simulink model "QueuingSys"  (R2019a)
settings: Solver=VariableStepAuto  StartTime=0.0  StopTime=100  RelTol=1e-3  EnableMultiTasking=on
undefined symbols (not defined in the file or in its folder): m, n
(part 2 of 5)

== system QueuingSys/Server18 ==
  Entity Generator1 : EntityGenerator  OutputPortMessageModes=m  TimeSource=MATLAB action  IntergenerationTimeAction=dt =MMPPArrivalTime35();  EntityType=Structured  EntityTypeName=Entity
  Entity Queue1 : EntityQueue  InputPortMessageModes=m  OutputPortMessageModes=m  Capacity=Inf  MulticastTag=B
      settings: OutputPortMap=o5
  Entity Server : EntityServer  InputPortMessageModes=m  OutputPortMessageModes=m  Capacity=2  ServiceTimeSource=MATLAB action  ServiceTimeAction=dt =MMPPArrivalTime36();
  OS : EntityOutputSwitch  InputPortMessageModes=m  OutputPortMessageModes=m,m,m,m,m,m,m,m,m,m,m,m,m,m,m,m,m,m,m,m  NumberOutputPorts=20  SwitchingCriterion=Round robin  SwitchAttributeName=Attribute1
      settings: OutputPortMap=o0,o1,o2,o3,o4,o5,o6,o7,o8,o9,o10,o11,o12,o13,o14,o15,o16,o17,o18,o19
  tag scope: Goto18_10=global, Goto18_11=global, Goto18_12=global, Goto18_13=global, Goto18_14=global, Goto18_15=global, Goto18_16=global, Goto18_17=global, Goto18_18=global, Goto18_19=global, Goto18_1=global, Goto18_20=global, Goto18_2=global, Goto18_3=global, Goto18_4=global, Goto18_5=global, Goto18_6=global, Goto18_7=global, Goto18_8=global, Goto18_9=global
  wires:
  Entity Queue1/1 -> Entity Server/1
  Entity Generator1/1 -> Entity Queue1/1
  Entity Server/1 -> OS/1
  OS/1 -> [Goto18_1]
  OS/2 -> [Goto18_2]
  OS/3 -> [Goto18_3]
  OS/4 -> [Goto18_4]
  OS/5 -> [Goto18_5]
  OS/6 -> [Goto18_6]
  OS/7 -> [Goto18_7]
  OS/8 -> [Goto18_8]
  OS/9 -> [Goto18_9]
  OS/10 -> [Goto18_10]
  OS/11 -> [Goto18_11]
  OS/12 -> [Goto18_12]
  OS/13 -> [Goto18_13]
  OS/14 -> [Goto18_14]
  OS/15 -> [Goto18_15]
  OS/16 -> [Goto18_16]
  OS/17 -> [Goto18_17]
  OS/18 -> [Goto18_18]
  OS/19 -> [Goto18_19]
  OS/20 -> [Goto18_20]

== system QueuingSys/Server19 ==
  Entity Generator1 : EntityGenerator  OutputPortMessageModes=m  TimeSource=MATLAB action  IntergenerationTimeAction=dt =MMPPArrivalTime37();  EntityType=Structured  EntityTypeName=Entity
  Entity Queue1 : EntityQueue  InputPortMessageModes=m  OutputPortMessageModes=m  Capacity=Inf  MulticastTag=B
      settings: OutputPortMap=o5
  Entity Server : EntityServer  InputPortMessageModes=m  OutputPortMessageModes=m  Capacity=3  ServiceTimeSource=MATLAB action  ServiceTimeAction=dt =MMPPArrivalTime38();
  OS : EntityOutputSwitch  InputPortMessageModes=m  OutputPortMessageModes=m,m,m,m,m,m,m,m,m,m,m,m,m,m,m,m,m,m,m,m  NumberOutputPorts=20  SwitchingCriterion=Round robin  SwitchAttributeName=Attribute1
      settings: OutputPortMap=o0,o1,o2,o3,o4,o5,o6,o7,o8,o9,o10,o11,o12,o13,o14,o15,o16,o17,o18,o19
  tag scope: Goto19_10=global, Goto19_11=global, Goto19_12=global, Goto19_13=global, Goto19_14=global, Goto19_15=global, Goto19_16=global, Goto19_17=global, Goto19_18=global, Goto19_19=global, Goto19_1=global, Goto19_20=global, Goto19_2=global, Goto19_3=global, Goto19_4=global, Goto19_5=global, Goto19_6=global, Goto19_7=global, Goto19_8=global, Goto19_9=global
  wires:
  Entity Server/1 -> OS/1
  Entity Generator1/1 -> Entity Queue1/1
  Entity Queue1/1 -> Entity Server/1
  OS/1 -> [Goto19_1]
  OS/2 -> [Goto19_2]
  OS/3 -> [Goto19_3]
  OS/4 -> [Goto19_4]
  OS/5 -> [Goto19_5]
  OS/6 -> [Goto19_6]
  OS/7 -> [Goto19_7]
  OS/8 -> [Goto19_8]
  OS/9 -> [Goto19_9]
  OS/10 -> [Goto19_10]
  OS/11 -> [Goto19_11]
  OS/12 -> [Goto19_12]
  OS/13 -> [Goto19_13]
  OS/14 -> [Goto19_14]
  OS/15 -> [Goto19_15]
  OS/16 -> [Goto19_16]
  OS/17 -> [Goto19_17]
  OS/18 -> [Goto19_18]
  OS/19 -> [Goto19_19]
  OS/20 -> [Goto19_20]

== system QueuingSys/Server2 ==
  Entity Generator1 : EntityGenerator  OutputPortMessageModes=m  TimeSource=MATLAB action  IntergenerationTimeAction=dt =MMPPArrivalTime3();  EntityType=Structured  EntityTypeName=Entity
  Entity Queue1 : EntityQueue  InputPortMessageModes=m  OutputPortMessageModes=m  Capacity=Inf  MulticastTag=B
      settings: OutputPortMap=o5
  Entity Server : EntityServer  InputPortMessageModes=m  OutputPortMessageModes=m  Capacity=1  ServiceTimeSource=MATLAB action  ServiceTimeAction=dt =MMPPArrivalTime4();
  OS : EntityOutputSwitch  InputPortMessageModes=m  OutputPortMessageModes=m,m,m,m,m,m,m,m,m,m,m,m,m,m,m,m,m,m,m,m  NumberOutputPorts=20  SwitchingCriterion=Round robin  SwitchAttributeName=Attribute1
      settings: OutputPortMap=o0,o1,o2,o3,o4,o5,o6,o7,o8,o9,o10,o11,o12,o13,o14,o15,o16,o17,o18,o19
  tag scope: Goto2_10=global, Goto2_11=global, Goto2_12=global, Goto2_13=global, Goto2_14=global, Goto2_15=global, Goto2_16=global, Goto2_17=global, Goto2_18=global, Goto2_19=global, Goto2_1=global, Goto2_20=global, Goto2_2=global, Goto2_3=global, Goto2_4=global, Goto2_5=global, Goto2_6=global, Goto2_7=global, Goto2_8=global, Goto2_9=global
  wires:
  Entity Queue1/1 -> Entity Server/1
  Entity Generator1/1 -> Entity Queue1/1
  Entity Server/1 -> OS/1
  OS/1 -> [Goto2_1]
  OS/2 -> [Goto2_2]
  OS/3 -> [Goto2_3]
  OS/4 -> [Goto2_4]
  OS/5 -> [Goto2_5]
  OS/6 -> [Goto2_6]
  OS/7 -> [Goto2_7]
  OS/8 -> [Goto2_8]
  OS/9 -> [Goto2_9]
  OS/10 -> [Goto2_10]
  OS/11 -> [Goto2_11]
  OS/12 -> [Goto2_12]
  OS/13 -> [Goto2_13]
  OS/14 -> [Goto2_14]
  OS/15 -> [Goto2_15]
  OS/16 -> [Goto2_16]
  OS/17 -> [Goto2_17]
  OS/18 -> [Goto2_18]
  OS/19 -> [Goto2_19]
  OS/20 -> [Goto2_20]

== system QueuingSys/Server20 ==
  Entity Generator1 : EntityGenerator  OutputPortMessageModes=m  TimeSource=MATLAB action  IntergenerationTimeAction=dt =MMPPArrivalTime39();  EntityType=Structured  EntityTypeName=Entity
  Entity Queue1 : EntityQueue  InputPortMessageModes=m  OutputPortMessageModes=m  Capacity=Inf  MulticastTag=B
      settings: OutputPortMap=o5
  Entity Server : EntityServer  InputPortMessageModes=m  OutputPortMessageModes=m  Capacity=3  ServiceTimeSource=MATLAB action  ServiceTimeAction=dt =MMPPArrivalTime40();
  OS : EntityOutputSwitch  InputPortMessageModes=m  OutputPortMessageModes=m,m,m,m,m,m,m,m,m,m,m,m,m,m,m,m,m,m,m,m  NumberOutputPorts=20  SwitchingCriterion=Round robin  SwitchAttributeName=Attribute1
      settings: OutputPortMap=o0,o1,o2,o3,o4,o5,o6,o7,o8,o9,o10,o11,o12,o13,o14,o15,o16,o17,o18,o19
  tag scope: Goto20_10=global, Goto20_11=global, Goto20_12=global, Goto20_13=global, Goto20_14=global, Goto20_15=global, Goto20_16=global, Goto20_17=global, Goto20_18=global, Goto20_19=global, Goto20_1=global, Goto20_20=global, Goto20_2=global, Goto20_3=global, Goto20_4=global, Goto20_5=global, Goto20_6=global, Goto20_7=global, Goto20_8=global, Goto20_9=global
  wires:
  Entity Queue1/1 -> Entity Server/1
  Entity Generator1/1 -> Entity Queue1/1
  Entity Server/1 -> OS/1
  OS/1 -> [Goto20_1]
  OS/2 -> [Goto20_2]
  OS/3 -> [Goto20_3]
  OS/4 -> [Goto20_4]
  OS/5 -> [Goto20_5]
  OS/6 -> [Goto20_6]
  OS/7 -> [Goto20_7]
  OS/8 -> [Goto20_8]
  OS/9 -> [Goto20_9]
  OS/10 -> [Goto20_10]
  OS/11 -> [Goto20_11]
  OS/12 -> [Goto20_12]
  OS/13 -> [Goto20_13]
  OS/14 -> [Goto20_14]
  OS/15 -> [Goto20_15]
  OS/16 -> [Goto20_16]
  OS/17 -> [Goto20_17]
  OS/18 -> [Goto20_18]
  OS/19 -> [Goto20_19]
  OS/20 -> [Goto20_20]

== system QueuingSys/Server21 ==
  Entity Generator1 : EntityGenerator  OutputPortMessageModes=m  TimeSource=MATLAB action  IntergenerationTimeAction=dt =MMPPArrivalTime41();  EntityType=Structured  EntityTypeName=Entity
  Entity Queue1 : EntityQueue  InputPortMessageModes=m  OutputPortMessageModes=m  Capacity=Inf  MulticastTag=B
      settings: OutputPortMap=o5
  Entity Server : EntityServer  InputPortMessageModes=m  OutputPortMessageModes=m  Capacity=2  ServiceTimeSource=MATLAB action  ServiceTimeAction=dt =MMPPArrivalTime42();
  OS : EntityOutputSwitch  InputPortMessageModes=m  OutputPortMessageModes=m,m,m,m,m,m,m,m,m,m,m,m,m,m,m,m,m,m,m,m  NumberOutputPorts=20  SwitchingCriterion=Round robin  SwitchAttributeName=Attribute1
      settings: OutputPortMap=o0,o1,o2,o3,o4,o5,o6,o7,o8,o9,o10,o11,o12,o13,o14,o15,o16,o17,o18,o19
  tag scope: Goto21_10=global, Goto21_11=global, Goto21_12=global, Goto21_13=global, Goto21_14=global, Goto21_15=global, Goto21_16=global, Goto21_17=global, Goto21_18=global, Goto21_19=global, Goto21_1=global, Goto21_20=global, Goto21_2=global, Goto21_3=global, Goto21_4=global, Goto21_5=global, Goto21_6=global, Goto21_7=global, Goto21_8=global, Goto21_9=global
  wires:
  Entity Server/1 -> OS/1
  Entity Generator1/1 -> Entity Queue1/1
  Entity Queue1/1 -> Entity Server/1
  OS/1 -> [Goto21_1]
  OS/2 -> [Goto21_2]
  OS/3 -> [Goto21_3]
  OS/4 -> [Goto21_4]
  OS/5 -> [Goto21_5]
  OS/6 -> [Goto21_6]
  OS/7 -> [Goto21_7]
  OS/8 -> [Goto21_8]
  OS/9 -> [Goto21_9]
  OS/10 -> [Goto21_10]
  OS/11 -> [Goto21_11]
  OS/12 -> [Goto21_12]
  OS/13 -> [Goto21_13]
  OS/14 -> [Goto21_14]
  OS/15 -> [Goto21_15]
  OS/16 -> [Goto21_16]
  OS/17 -> [Goto21_17]
  OS/18 -> [Goto21_18]
  OS/19 -> [Goto21_19]
  OS/20 -> [Goto21_20]

== system QueuingSys/Server22 ==
  Entity Generator1 : EntityGenerator  OutputPortMessageModes=m  TimeSource=MATLAB action  IntergenerationTimeAction=dt =MMPPArrivalTime43();  EntityType=Structured  EntityTypeName=Entity
  Entity Queue1 : EntityQueue  InputPortMessageModes=m  OutputPortMessageModes=m  Capacity=Inf  MulticastTag=B
      settings: OutputPortMap=o5
  Entity Server : EntityServer  InputPortMessageModes=m  OutputPortMessageModes=m  ServiceTimeSource=MATLAB action  ServiceTimeAction=dt =MMPPArrivalTime44();
  OS : EntityOutputSwitch  InputPortMessageModes=m  OutputPortMessageModes=m,m,m,m,m,m,m,m,m,m,m,m,m,m,m,m,m,m,m,m  NumberOutputPorts=20  SwitchingCriterion=Round robin  SwitchAttributeName=Attribute1
      settings: OutputPortMap=o0,o1,o2,o3,o4,o5,o6,o7,o8,o9,o10,o11,o12,o13,o14,o15,o16,o17,o18,o19
  tag scope: Goto22_10=global, Goto22_11=global, Goto22_12=global, Goto22_13=global, Goto22_14=global, Goto22_15=global, Goto22_16=global, Goto22_17=global, Goto22_18=global, Goto22_19=global, Goto22_1=global, Goto22_20=global, Goto22_2=global, Goto22_3=global, Goto22_4=global, Goto22_5=global, Goto22_6=global, Goto22_7=global, Goto22_8=global, Goto22_9=global
  wires:
  Entity Queue1/1 -> Entity Server/1
  Entity Generator1/1 -> Entity Queue1/1
  Entity Server/1 -> OS/1
  OS/1 -> [Goto22_1]
  OS/2 -> [Goto22_2]
  OS/3 -> [Goto22_3]
  OS/4 -> [Goto22_4]
  OS/5 -> [Goto22_5]
  OS/6 -> [Goto22_6]
  OS/7 -> [Goto22_7]
  OS/8 -> [Goto22_8]
  OS/9 -> [Goto22_9]
  OS/10 -> [Goto22_10]
  OS/11 -> [Goto22_11]
  OS/12 -> [Goto22_12]
  OS/13 -> [Goto22_13]
  OS/14 -> [Goto22_14]
  OS/15 -> [Goto22_15]
  OS/16 -> [Goto22_16]
  OS/17 -> [Goto22_17]
  OS/18 -> [Goto22_18]
  OS/19 -> [Goto22_19]
  OS/20 -> [Goto22_20]

== system QueuingSys/Server23 ==
  Entity Generator1 : EntityGenerator  OutputPortMessageModes=m  TimeSource=MATLAB action  IntergenerationTimeAction=dt =MMPPArrivalTime45();  EntityType=Structured  EntityTypeName=Entity
  Entity Queue1 : EntityQueue  InputPortMessageModes=m  OutputPortMessageModes=m  Capacity=Inf  MulticastTag=B
      settings: OutputPortMap=o5
  Entity Server : EntityServer  InputPortMessageModes=m  OutputPortMessageModes=m  Capacity=7  ServiceTimeSource=MATLAB action  ServiceTimeAction=dt =MMPPArrivalTime46();
  OS : EntityOutputSwitch  InputPortMessageModes=m  OutputPortMessageModes=m,m,m,m,m,m,m,m,m,m,m,m,m,m,m,m,m,m,m,m  NumberOutputPorts=20  SwitchingCriterion=Round robin  SwitchAttributeName=Attribute1
      settings: OutputPortMap=o0,o1,o2,o3,o4,o5,o6,o7,o8,o9,o10,o11,o12,o13,o14,o15,o16,o17,o18,o19
  tag scope: Goto23_10=global, Goto23_11=global, Goto23_12=global, Goto23_13=global, Goto23_14=global, Goto23_15=global, Goto23_16=global, Goto23_17=global, Goto23_18=global, Goto23_19=global, Goto23_1=global, Goto23_20=global, Goto23_2=global, Goto23_3=global, Goto23_4=global, Goto23_5=global, Goto23_6=global, Goto23_7=global, Goto23_8=global, Goto23_9=global
  wires:
  Entity Server/1 -> OS/1
  Entity Generator1/1 -> Entity Queue1/1
  Entity Queue1/1 -> Entity Server/1
  OS/1 -> [Goto23_1]
  OS/2 -> [Goto23_2]
  OS/3 -> [Goto23_3]
  OS/4 -> [Goto23_4]
  OS/5 -> [Goto23_5]
  OS/6 -> [Goto23_6]
  OS/7 -> [Goto23_7]
  OS/8 -> [Goto23_8]
  OS/9 -> [Goto23_9]
  OS/10 -> [Goto23_10]
  OS/11 -> [Goto23_11]
  OS/12 -> [Goto23_12]
  OS/13 -> [Goto23_13]
  OS/14 -> [Goto23_14]
  OS/15 -> [Goto23_15]
  OS/16 -> [Goto23_16]
  OS/17 -> [Goto23_17]
  OS/18 -> [Goto23_18]
  OS/19 -> [Goto23_19]
  OS/20 -> [Goto23_20]

== system QueuingSys/Server24 ==
  Entity Generator1 : EntityGenerator  OutputPortMessageModes=m  TimeSource=MATLAB action  IntergenerationTimeAction=dt =MMPPArrivalTime47();  EntityType=Structured  EntityTypeName=Entity
  Entity Queue1 : EntityQueue  InputPortMessageModes=m  OutputPortMessageModes=m  Capacity=Inf  MulticastTag=B
      settings: OutputPortMap=o5
  Entity Server : EntityServer  InputPortMessageModes=m  OutputPortMessageModes=m  Capacity=4  ServiceTimeSource=MATLAB action  ServiceTimeAction=dt =MMPPArrivalTime48();
  OS : EntityOutputSwitch  InputPortMessageModes=m  OutputPortMessageModes=m,m,m,m,m,m,m,m,m,m,m,m,m,m,m,m,m,m,m,m  NumberOutputPorts=20  SwitchingCriterion=Round robin  SwitchAttributeName=Attribute1
      settings: OutputPortMap=o0,o1,o2,o3,o4,o5,o6,o7,o8,o9,o10,o11,o12,o13,o14,o15,o16,o17,o18,o19
  tag scope: Goto24_10=global, Goto24_11=global, Goto24_12=global, Goto24_13=global, Goto24_14=global, Goto24_15=global, Goto24_16=global, Goto24_17=global, Goto24_18=global, Goto24_19=global, Goto24_1=global, Goto24_20=global, Goto24_2=global, Goto24_3=global, Goto24_4=global, Goto24_5=global, Goto24_6=global, Goto24_7=global, Goto24_8=global, Goto24_9=global
  wires:
  Entity Queue1/1 -> Entity Server/1
  Entity Generator1/1 -> Entity Queue1/1
  Entity Server/1 -> OS/1
  OS/1 -> [Goto24_1]
  OS/2 -> [Goto24_2]
  OS/3 -> [Goto24_3]
  OS/4 -> [Goto24_4]
  OS/5 -> [Goto24_5]
  OS/6 -> [Goto24_6]
  OS/7 -> [Goto24_7]
  OS/8 -> [Goto24_8]
  OS/9 -> [Goto24_9]
  OS/10 -> [Goto24_10]
  OS/11 -> [Goto24_11]
  OS/12 -> [Goto24_12]
  OS/13 -> [Goto24_13]
  OS/14 -> [Goto24_14]
  OS/15 -> [Goto24_15]
  OS/16 -> [Goto24_16]
  OS/17 -> [Goto24_17]
  OS/18 -> [Goto24_18]
  OS/19 -> [Goto24_19]
  OS/20 -> [Goto24_20]

== system QueuingSys/Server25 ==
  Entity Generator1 : EntityGenerator  OutputPortMessageModes=m  TimeSource=MATLAB action  IntergenerationTimeAction=dt =MMPPArrivalTime49();  EntityType=Structured  EntityTypeName=Entity
  Entity Queue1 : EntityQueue  InputPortMessageModes=m  OutputPortMessageModes=m  Capacity=Inf  MulticastTag=B
      settings: OutputPortMap=o5
  Entity Server : EntityServer  InputPortMessageModes=m  OutputPortMessageModes=m  Capacity=6  ServiceTimeSource=MATLAB action  ServiceTimeAction=dt =MMPPArrivalTime50();
  OS : EntityOutputSwitch  InputPortMessageModes=m  OutputPortMessageModes=m,m,m,m,m,m,m,m,m,m,m,m,m,m,m,m,m,m,m,m  NumberOutputPorts=20  SwitchingCriterion=Round robin  SwitchAttributeName=Attribute1
      settings: OutputPortMap=o0,o1,o2,o3,o4,o5,o6,o7,o8,o9,o10,o11,o12,o13,o14,o15,o16,o17,o18,o19
  tag scope: Goto25_10=global, Goto25_11=global, Goto25_12=global, Goto25_13=global, Goto25_14=global, Goto25_15=global, Goto25_16=global, Goto25_17=global, Goto25_18=global, Goto25_19=global, Goto25_1=global, Goto25_20=global, Goto25_2=global, Goto25_3=global, Goto25_4=global, Goto25_5=global, Goto25_6=global, Goto25_7=global, Goto25_8=global, Goto25_9=global
  wires:
  Entity Server/1 -> OS/1
  Entity Generator1/1 -> Entity Queue1/1
  Entity Queue1/1 -> Entity Server/1
  OS/1 -> [Goto25_1]
  OS/2 -> [Goto25_2]
  OS/3 -> [Goto25_3]
  OS/4 -> [Goto25_4]
  OS/5 -> [Goto25_5]
  OS/6 -> [Goto25_6]
  OS/7 -> [Goto25_7]
  OS/8 -> [Goto25_8]
  OS/9 -> [Goto25_9]
  OS/10 -> [Goto25_10]
  OS/11 -> [Goto25_11]
  OS/12 -> [Goto25_12]
  OS/13 -> [Goto25_13]
  OS/14 -> [Goto25_14]
  OS/15 -> [Goto25_15]
  OS/16 -> [Goto25_16]
  OS/17 -> [Goto25_17]
  OS/18 -> [Goto25_18]
  OS/19 -> [Goto25_19]
  OS/20 -> [Goto25_20]

== system QueuingSys/Server3 ==
  Entity Generator1 : EntityGenerator  OutputPortMessageModes=m  TimeSource=MATLAB action  IntergenerationTimeAction=dt =MMPPArrivalTime5();  EntityType=Structured  EntityTypeName=Entity
  Entity Queue1 : EntityQueue  InputPortMessageModes=m  OutputPortMessageModes=m  Capacity=Inf  MulticastTag=B
      settings: OutputPortMap=o5
  Entity Server : EntityServer  InputPortMessageModes=m  OutputPortMessageModes=m  Capacity=3  ServiceTimeSource=MATLAB action  ServiceTimeAction=dt =MMPPArrivalTime6();
  OS : EntityOutputSwitch  InputPortMessageModes=m  OutputPortMessageModes=m,m,m,m,m,m,m,m,m,m,m,m,m,m,m,m,m,m,m,m  NumberOutputPorts=20  SwitchingCriterion=Round robin  SwitchAttributeName=Attribute1
      settings: OutputPortMap=o0,o1,o2,o3,o4,o5,o6,o7,o8,o9,o10,o11,o12,o13,o14,o15,o16,o17,o18,o19
  tag scope: Goto3_10=global, Goto3_11=global, Goto3_12=global, Goto3_13=global, Goto3_14=global, Goto3_15=global, Goto3_16=global, Goto3_17=global, Goto3_18=global, Goto3_19=global, Goto3_1=global, Goto3_20=global, Goto3_2=global, Goto3_3=global, Goto3_4=global, Goto3_5=global, Goto3_6=global, Goto3_7=global, Goto3_8=global, Goto3_9=global
  wires:
  Entity Server/1 -> OS/1
  Entity Generator1/1 -> Entity Queue1/1
  Entity Queue1/1 -> Entity Server/1
  OS/1 -> [Goto3_1]
  OS/2 -> [Goto3_2]
  OS/3 -> [Goto3_3]
  OS/4 -> [Goto3_4]
  OS/5 -> [Goto3_5]
  OS/6 -> [Goto3_6]
  OS/7 -> [Goto3_7]
  OS/8 -> [Goto3_8]
  OS/9 -> [Goto3_9]
  OS/10 -> [Goto3_10]
  OS/11 -> [Goto3_11]
  OS/12 -> [Goto3_12]
  OS/13 -> [Goto3_13]
  OS/14 -> [Goto3_14]
  OS/15 -> [Goto3_15]
  OS/16 -> [Goto3_16]
  OS/17 -> [Goto3_17]
  OS/18 -> [Goto3_18]
  OS/19 -> [Goto3_19]
  OS/20 -> [Goto3_20]

== system QueuingSys/Server4 ==
  Entity Generator1 : EntityGenerator  OutputPortMessageModes=m  TimeSource=MATLAB action  IntergenerationTimeAction=dt =MMPPArrivalTime7();  EntityType=Structured  EntityTypeName=Entity
  Entity Queue1 : EntityQueue  InputPortMessageModes=m  OutputPortMessageModes=m  Capacity=Inf  MulticastTag=B
      settings: OutputPortMap=o5
  Entity Server : EntityServer  InputPortMessageModes=m  OutputPortMessageModes=m  Capacity=1  ServiceTimeSource=MATLAB action  ServiceTimeAction=dt =MMPPArrivalTime8();
  OS : EntityOutputSwitch  InputPortMessageModes=m  OutputPortMessageModes=m,m,m,m,m,m,m,m,m,m,m,m,m,m,m,m,m,m,m,m  NumberOutputPorts=20  SwitchingCriterion=Round robin  SwitchAttributeName=Attribute1
      settings: OutputPortMap=o0,o1,o2,o3,o4,o5,o6,o7,o8,o9,o10,o11,o12,o13,o14,o15,o16,o17,o18,o19
  tag scope: Goto4_10=global, Goto4_11=global, Goto4_12=global, Goto4_13=global, Goto4_14=global, Goto4_15=global, Goto4_16=global, Goto4_17=global, Goto4_18=global, Goto4_19=global, Goto4_1=global, Goto4_20=global, Goto4_2=global, Goto4_3=global, Goto4_4=global, Goto4_5=global, Goto4_6=global, Goto4_7=global, Goto4_8=global, Goto4_9=global
  wires:
  Entity Queue1/1 -> Entity Server/1
  Entity Generator1/1 -> Entity Queue1/1
  Entity Server/1 -> OS/1
  OS/1 -> [Goto4_1]
  OS/2 -> [Goto4_2]
  OS/3 -> [Goto4_3]
  OS/4 -> [Goto4_4]
  OS/5 -> [Goto4_5]
  OS/6 -> [Goto4_6]
  OS/7 -> [Goto4_7]
  OS/8 -> [Goto4_8]
  OS/9 -> [Goto4_9]
  OS/10 -> [Goto4_10]
  OS/11 -> [Goto4_11]
  OS/12 -> [Goto4_12]
  OS/13 -> [Goto4_13]
  OS/14 -> [Goto4_14]
  OS/15 -> [Goto4_15]
  OS/16 -> [Goto4_16]
  OS/17 -> [Goto4_17]
  OS/18 -> [Goto4_18]
  OS/19 -> [Goto4_19]
  OS/20 -> [Goto4_20]

== system QueuingSys/Server5 ==
  Entity Generator1 : EntityGenerator  OutputPortMessageModes=m  TimeSource=MATLAB action  IntergenerationTimeAction=dt =MMPPArrivalTime9();  EntityType=Structured  EntityTypeName=Entity
  Entity Queue1 : EntityQueue  InputPortMessageModes=m  OutputPortMessageModes=m  Capacity=Inf  MulticastTag=B
      settings: OutputPortMap=o5
  Entity Server : EntityServer  InputPortMessageModes=m  OutputPortMessageModes=m  Capacity=6  ServiceTimeSource=MATLAB action  ServiceTimeAction=dt =MMPPArrivalTime10();
  OS : EntityOutputSwitch  InputPortMessageModes=m  OutputPortMessageModes=m,m,m,m,m,m,m,m,m,m,m,m,m,m,m,m,m,m,m,m  NumberOutputPorts=20  SwitchingCriterion=Round robin  SwitchAttributeName=Attribute1
      settings: OutputPortMap=o0,o1,o2,o3,o4,o5,o6,o7,o8,o9,o10,o11,o12,o13,o14,o15,o16,o17,o18,o19
  tag scope: Goto5_10=global, Goto5_11=global, Goto5_12=global, Goto5_13=global, Goto5_14=global, Goto5_15=global, Goto5_16=global, Goto5_17=global, Goto5_18=global, Goto5_19=global, Goto5_1=global, Goto5_20=global, Goto5_2=global, Goto5_3=global, Goto5_4=global, Goto5_5=global, Goto5_6=global, Goto5_7=global, Goto5_8=global, Goto5_9=global
  wires:
  Entity Server/1 -> OS/1
  Entity Generator1/1 -> Entity Queue1/1
  Entity Queue1/1 -> Entity Server/1
  OS/1 -> [Goto5_1]
  OS/2 -> [Goto5_2]
  OS/3 -> [Goto5_3]
  OS/4 -> [Goto5_4]
  OS/5 -> [Goto5_5]
  OS/6 -> [Goto5_6]
  OS/7 -> [Goto5_7]
  OS/8 -> [Goto5_8]
  OS/9 -> [Goto5_9]
  OS/10 -> [Goto5_10]
  OS/11 -> [Goto5_11]
  OS/12 -> [Goto5_12]
  OS/13 -> [Goto5_13]
  OS/14 -> [Goto5_14]
  OS/15 -> [Goto5_15]
  OS/16 -> [Goto5_16]
  OS/17 -> [Goto5_17]
  OS/18 -> [Goto5_18]
  OS/19 -> [Goto5_19]
  OS/20 -> [Goto5_20]

== system QueuingSys/Server6 ==
  Entity Generator1 : EntityGenerator  OutputPortMessageModes=m  TimeSource=MATLAB action  IntergenerationTimeAction=dt =MMPPArrivalTime11();  EntityType=Structured  EntityTypeName=Entity
  Entity Queue1 : EntityQueue  InputPortMessageModes=m  OutputPortMessageModes=m  Capacity=Inf  MulticastTag=B
      settings: OutputPortMap=o5
  Entity Server : EntityServer  InputPortMessageModes=m  OutputPortMessageModes=m  Capacity=3  ServiceTimeSource=MATLAB action  ServiceTimeAction=dt =MMPPArrivalTime12();
  OS : EntityOutputSwitch  InputPortMessageModes=m  OutputPortMessageModes=m,m,m,m,m,m,m,m,m,m,m,m,m,m,m,m,m,m,m,m  NumberOutputPorts=20  SwitchingCriterion=Round robin  SwitchAttributeName=Attribute1
      settings: OutputPortMap=o0,o1,o2,o3,o4,o5,o6,o7,o8,o9,o10,o11,o12,o13,o14,o15,o16,o17,o18,o19
  tag scope: Goto6_10=global, Goto6_11=global, Goto6_12=global, Goto6_13=global, Goto6_14=global, Goto6_15=global, Goto6_16=global, Goto6_17=global, Goto6_18=global, Goto6_19=global, Goto6_1=global, Goto6_20=global, Goto6_2=global, Goto6_3=global, Goto6_4=global, Goto6_5=global, Goto6_6=global, Goto6_7=global, Goto6_8=global, Goto6_9=global
  wires:
  Entity Queue1/1 -> Entity Server/1
  Entity Generator1/1 -> Entity Queue1/1
  Entity Server/1 -> OS/1
  OS/1 -> [Goto6_1]
  OS/2 -> [Goto6_2]
  OS/3 -> [Goto6_3]
  OS/4 -> [Goto6_4]
  OS/5 -> [Goto6_5]
  OS/6 -> [Goto6_6]
  OS/7 -> [Goto6_7]
  OS/8 -> [Goto6_8]
  OS/9 -> [Goto6_9]
  OS/10 -> [Goto6_10]
  OS/11 -> [Goto6_11]
  OS/12 -> [Goto6_12]
  OS/13 -> [Goto6_13]
  OS/14 -> [Goto6_14]
  OS/15 -> [Goto6_15]
  OS/16 -> [Goto6_16]
  OS/17 -> [Goto6_17]
  OS/18 -> [Goto6_18]
  OS/19 -> [Goto6_19]
  OS/20 -> [Goto6_20]

== system QueuingSys/Server7 ==
  Entity Generator1 : EntityGenerator  OutputPortMessageModes=m  TimeSource=MATLAB action  IntergenerationTimeAction=dt =MMPPArrivalTime13();  EntityType=Structured  EntityTypeName=Entity
  Entity Queue1 : EntityQueue  InputPortMessageModes=m  OutputPortMessageModes=m  Capacity=Inf  MulticastTag=B
      settings: OutputPortMap=o5
  Entity Server : EntityServer  InputPortMessageModes=m  OutputPortMessageModes=m  Capacity=4  ServiceTimeSource=MATLAB action  ServiceTimeAction=dt =MMPPArrivalTime14();
  OS : EntityOutputSwitch  InputPortMessageModes=m  OutputPortMessageModes=m,m,m,m,m,m,m,m,m,m,m,m,m,m,m,m,m,m,m,m  NumberOutputPorts=20  SwitchingCriterion=Round robin  SwitchAttributeName=Attribute1
      settings: OutputPortMap=o0,o1,o2,o3,o4,o5,o6,o7,o8,o9,o10,o11,o12,o13,o14,o15,o16,o17,o18,o19
  tag scope: Goto7_10=global, Goto7_11=global, Goto7_12=global, Goto7_13=global, Goto7_14=global, Goto7_15=global, Goto7_16=global, Goto7_17=global, Goto7_18=global, Goto7_19=global, Goto7_1=global, Goto7_20=global, Goto7_2=global, Goto7_3=global, Goto7_4=global, Goto7_5=global, Goto7_6=global, Goto7_7=global, Goto7_8=global, Goto7_9=global
  wires:
  Entity Server/1 -> OS/1
  Entity Generator1/1 -> Entity Queue1/1
  Entity Queue1/1 -> Entity Server/1
  OS/1 -> [Goto7_1]
  OS/2 -> [Goto7_2]
  OS/3 -> [Goto7_3]
  OS/4 -> [Goto7_4]
  OS/5 -> [Goto7_5]
  OS/6 -> [Goto7_6]
  OS/7 -> [Goto7_7]
  OS/8 -> [Goto7_8]
  OS/9 -> [Goto7_9]
  OS/10 -> [Goto7_10]
  OS/11 -> [Goto7_11]
  OS/12 -> [Goto7_12]
  OS/13 -> [Goto7_13]
  OS/14 -> [Goto7_14]
  OS/15 -> [Goto7_15]
  OS/16 -> [Goto7_16]
  OS/17 -> [Goto7_17]
  OS/18 -> [Goto7_18]
  OS/19 -> [Goto7_19]
  OS/20 -> [Goto7_20]

== system QueuingSys/Server8 ==
  Entity Generator1 : EntityGenerator  OutputPortMessageModes=m  TimeSource=MATLAB action  IntergenerationTimeAction=dt =MMPPArrivalTime15();  EntityType=Structured  EntityTypeName=Entity
  Entity Queue1 : EntityQueue  InputPortMessageModes=m  OutputPortMessageModes=m  Capacity=Inf  MulticastTag=B
      settings: OutputPortMap=o5
  Entity Server : EntityServer  InputPortMessageModes=m  OutputPortMessageModes=m  Capacity=2  ServiceTimeSource=MATLAB action  ServiceTimeAction=dt =MMPPArrivalTime16();
  OS : EntityOutputSwitch  InputPortMessageModes=m  OutputPortMessageModes=m,m,m,m,m,m,m,m,m,m,m,m,m,m,m,m,m,m,m,m  NumberOutputPorts=20  SwitchingCriterion=Round robin  SwitchAttributeName=Attribute1
      settings: OutputPortMap=o0,o1,o2,o3,o4,o5,o6,o7,o8,o9,o10,o11,o12,o13,o14,o15,o16,o17,o18,o19
  tag scope: Goto8_10=global, Goto8_11=global, Goto8_12=global, Goto8_13=global, Goto8_14=global, Goto8_15=global, Goto8_16=global, Goto8_17=global, Goto8_18=global, Goto8_19=global, Goto8_1=global, Goto8_20=global, Goto8_2=global, Goto8_3=global, Goto8_4=global, Goto8_5=global, Goto8_6=global, Goto8_7=global, Goto8_8=global, Goto8_9=global
  wires:
  Entity Queue1/1 -> Entity Server/1
  Entity Generator1/1 -> Entity Queue1/1
  Entity Server/1 -> OS/1
  OS/1 -> [Goto8_1]
  OS/2 -> [Goto8_2]
  OS/3 -> [Goto8_3]
  OS/4 -> [Goto8_4]
  OS/5 -> [Goto8_5]
  OS/6 -> [Goto8_6]
  OS/7 -> [Goto8_7]
  OS/8 -> [Goto8_8]
  OS/9 -> [Goto8_9]
  OS/10 -> [Goto8_10]
  OS/11 -> [Goto8_11]
  OS/12 -> [Goto8_12]
  OS/13 -> [Goto8_13]
  OS/14 -> [Goto8_14]
  OS/15 -> [Goto8_15]
  OS/16 -> [Goto8_16]
  OS/17 -> [Goto8_17]
  OS/18 -> [Goto8_18]
  OS/19 -> [Goto8_19]
  OS/20 -> [Goto8_20]

== system QueuingSys/Server9 ==
  Entity Generator1 : EntityGenerator  OutputPortMessageModes=m  TimeSource=MATLAB action  IntergenerationTimeAction=dt =MMPPArrivalTime17();  EntityType=Structured  EntityTypeName=Entity
  Entity Queue1 : EntityQueue  InputPortMessageModes=m  OutputPortMessageModes=m  Capacity=Inf  MulticastTag=B
      settings: OutputPortMap=o5
  Entity Server : EntityServer  InputPortMessageModes=m  OutputPortMessageModes=m  Capacity=6  ServiceTimeSource=MATLAB action  ServiceTimeAction=dt =MMPPArrivalTime18();
  OS : EntityOutputSwitch  InputPortMessageModes=m  OutputPortMessageModes=m,m,m,m,m,m,m,m,m,m,m,m,m,m,m,m,m,m,m,m  NumberOutputPorts=20  SwitchingCriterion=Round robin  SwitchAttributeName=Attribute1
      settings: OutputPortMap=o0,o1,o2,o3,o4,o5,o6,o7,o8,o9,o10,o11,o12,o13,o14,o15,o16,o17,o18,o19
  tag scope: Goto9_10=global, Goto9_11=global, Goto9_12=global, Goto9_13=global, Goto9_14=global, Goto9_15=global, Goto9_16=global, Goto9_17=global, Goto9_18=global, Goto9_19=global, Goto9_1=global, Goto9_20=global, Goto9_2=global, Goto9_3=global, Goto9_4=global, Goto9_5=global, Goto9_6=global, Goto9_7=global, Goto9_8=global, Goto9_9=global
  wires:
  Entity Server/1 -> OS/1
  Entity Generator1/1 -> Entity Queue1/1
  Entity Queue1/1 -> Entity Server/1
  OS/1 -> [Goto9_1]
  OS/2 -> [Goto9_2]
  OS/3 -> [Goto9_3]
  OS/4 -> [Goto9_4]
  OS/5 -> [Goto9_5]
  OS/6 -> [Goto9_6]
  OS/7 -> [Goto9_7]
  OS/8 -> [Goto9_8]
  OS/9 -> [Goto9_9]
  OS/10 -> [Goto9_10]
  OS/11 -> [Goto9_11]
  OS/12 -> [Goto9_12]
  OS/13 -> [Goto9_13]
  OS/14 -> [Goto9_14]
  OS/15 -> [Goto9_15]
  OS/16 -> [Goto9_16]
  OS/17 -> [Goto9_17]
  OS/18 -> [Goto9_18]
  OS/19 -> [Goto9_19]
  OS/20 -> [Goto9_20]

== system QueuingSys/Distro/MMPPArrivalTime1 ==
  MMPPArrivalTime : TriggerPort  TriggerType=function-call  IsSimulinkFunction=on  FunctionName=MMPPArrivalTime1  VariantControl=Variant
  Constant : Constant  Value=[0.412159093658181 0.317831870182722 0.133931544933991 0.00987623758494989 0.0931069192135052 0.0330943344266506;0.163331203889296 0.00869673601137318 0.283742324915975 0.211971167379307 0.11317632270736 0.219082245096688;0.00212236020661071 0.193135683229019 0.00234252764520018 0.214233858159417 0.277978307809218 0.310187262950535;0.0541252967165364 0.159747585156857 0.187608310787008 0.254374469901602 0.0416620313631015 0.302482306074895;0.086209108981779 0.0915338902481286 0.121164620125895 0.260060432215067 0.141277614894353 0.299754333534778;0.0205315805580306 0.311905867627122 0.196157874483634 0.130236847543161 0.00863813726125668 0.332529692526796]  SampleTime=-1
  D : Memory  InitialCondition=[0.0621365072779505;0.77754382520324]  InheritSampleTime=on
  MMPP : MATLAB Function  TreatAsAtomicUnit=on
  Scope : Scope
  Scope1 : Scope
  T : Memory  InitialCondition=[0 0.883539674649741]  InheritSampleTime=on
  Uniform Random Number : UniformRandomNumber  Minimum=0  Seed=randi(5000)
  X : Memory  InitialCondition=1  InheritSampleTime=on
  t : ArgOut  DisableCoverage=on  ArgumentName=t
  wires:
  X/1 -> MMPP/1("x ")
  T/1 -> MMPP/2("T ")
  MMPP/2(T) -> T/1
  MMPP/4(t) -> t/1, Scope/1
  MMPP/1(x) -> X/1
  Constant/1 -> MMPP/4(M)
  Uniform Random Number/1 -> MMPP/5(rn)
  MMPP/3(D) -> D/1
  D/1 -> MMPP/3("D ")
  MMPP/5(lambda) -> Scope1/1

== system QueuingSys/Distro/MMPPArrivalTime10 ==
  MMPPArrivalTime : TriggerPort  TriggerType=function-call  IsSimulinkFunction=on  FunctionName=MMPPArrivalTime10  VariantControl=Variant
  Constant : Constant  Value=[0.14791658699818 0.189600378010944 0.0522305213407234 0.188296619056212 0.173178289859822 0.0661810030371976 0.182596601696922;0.0794053648880361 0.0641664402973216 0.132176652184913 0.0505924788278475 0.354867567711648 0.229506428771017 0.0892850673192174;0.000805645817566182 0.137377999930999 0.264390197221379 0.191194737152744 0.0775488147613002 0.224240672212579 0.104441932903432;0.0458057627295258 0.130302563675737 0.0116997460708938 0.148740821401665 0.236998414266189 0.332900857603768 0.0935518342522213;0.193138502331306 0.0989999748931925 0.19086977956625 0.0235469557245693 0.135948930153773 0.182564997567859 0.17493085976305;0.219770792720406 0.0192198470162457 0.120491618825333 0.160820548620779 0.293374803283644 0.163375970890363 0.0229464186432292;0.0343180300777731 0.0995286989280356 0.199816494653995 0.139200240722811 0.26610514025086 0.176275073861008 0.0847563215055173]  SampleTime=-1
  D : Memory  InitialCondition=[0.618966880542704;0.409787087237061]  InheritSampleTime=on
  MMPP : MATLAB Function  TreatAsAtomicUnit=on
  Scope : Scope
  Scope1 : Scope
  T : Memory  InitialCondition=[0 0.448845076916645]  InheritSampleTime=on
  Uniform Random Number : UniformRandomNumber  Minimum=0  Seed=randi(5000)
  X : Memory  InitialCondition=4  InheritSampleTime=on
  t : ArgOut  DisableCoverage=on  ArgumentName=t
  wires:
  MMPP/5(lambda) -> Scope1/1
  D/1 -> MMPP/3("D ")
  MMPP/3(D) -> D/1
  Uniform Random Number/1 -> MMPP/5(rn)
  Constant/1 -> MMPP/4(M)
  MMPP/1(x) -> X/1
  MMPP/4(t) -> Scope/1, t/1
  MMPP/2(T) -> T/1
  T/1 -> MMPP/2("T ")
  X/1 -> MMPP/1("x ")

== system QueuingSys/Distro/MMPPArrivalTime11 ==
  MMPPArrivalTime : TriggerPort  TriggerType=function-call  IsSimulinkFunction=on  FunctionName=MMPPArrivalTime11  VariantControl=Variant
  Constant : Constant  Value=[0.129047844835686 0.278956960252588 0.591995194911726;0.040407058542902 0.470518141853582 0.489074799603516;0.249192371895868 0.628688943715096 0.122118684389036]  SampleTime=-1
  D : Memory  InitialCondition=[0.0720193262477142;0.365845796787181]  InheritSampleTime=on
  MMPP : MATLAB Function  TreatAsAtomicUnit=on
  Scope : Scope
  Scope1 : Scope
  T : Memory  InitialCondition=[0 0.24115946512324]  InheritSampleTime=on
  Uniform Random Number : UniformRandomNumber  Minimum=0  Seed=randi(5000)
  X : Memory  InitialCondition=2  InheritSampleTime=on
  t : ArgOut  DisableCoverage=on  ArgumentName=t
  wires:
  MMPP/5(lambda) -> Scope1/1
  D/1 -> MMPP/3("D ")
  MMPP/3(D) -> D/1
  Uniform Random Number/1 -> MMPP/5(rn)
  Constant/1 -> MMPP/4(M)
  MMPP/1(x) -> X/1
  MMPP/4(t) -> Scope/1, t/1
  MMPP/2(T) -> T/1
  T/1 -> MMPP/2("T ")
  X/1 -> MMPP/1("x ")

== system QueuingSys/Distro/MMPPArrivalTime12 ==
  MMPPArrivalTime : TriggerPort  TriggerType=function-call  IsSimulinkFunction=on  FunctionName=MMPPArrivalTime12  VariantControl=Variant
  Constant : Constant  Value=[0.42033904731243 0.131944764480158 0.216711944818556 0.231004243388856;0.127158835766185 0.368738296302099 0.130640862813513 0.373462005118203;0.115344122895162 0.275606692894181 0.347350630331023 0.261698553879634;0.207647937806112 0.00582236608118863 0.443415410966499 0.343114285146201]  SampleTime=-1
  D : Memory  InitialCondition=[0.781345653172047;0.538427479061901]  InheritSampleTime=on
  MMPP : MATLAB Function  TreatAsAtomicUnit=on
  Scope : Scope
  Scope1 : Scope
  T : Memory  InitialCondition=[0 0.507848919116842]  InheritSampleTime=on
  Uniform Random Number : UniformRandomNumber  Minimum=0  Seed=randi(5000)
  X : Memory  InitialCondition=4  InheritSampleTime=on
  t : ArgOut  DisableCoverage=on  ArgumentName=t
  wires:
  MMPP/5(lambda) -> Scope1/1
  D/1 -> MMPP/3("D ")
  MMPP/3(D) -> D/1
  Uniform Random Number/1 -> MMPP/5(rn)
  Constant/1 -> MMPP/4(M)
  MMPP/1(x) -> X/1
  MMPP/4(t) -> Scope/1, t/1
  MMPP/2(T) -> T/1
  T/1 -> MMPP/2("T ")
  X/1 -> MMPP/1("x ")

== system QueuingSys/Distro/MMPPArrivalTime13 ==
  MMPPArrivalTime : TriggerPort  TriggerType=function-call  IsSimulinkFunction=on  FunctionName=MMPPArrivalTime13  VariantControl=Variant
  Constant : Constant  Value=[0.485145019468541 0.514854980531459;0.478032708696403 0.521967291303597]  SampleTime=-1
  D : Memory  InitialCondition=[0.667913624903703;0.502421972529354]  InheritSampleTime=on
  MMPP : MATLAB Function  TreatAsAtomicUnit=on
  Scope : Scope
  Scope1 : Scope
  T : Memory  InitialCondition=[0 0.359370267196457]  InheritSampleTime=on
  Uniform Random Number : UniformRandomNumber  Minimum=0  Seed=randi(5000)
  X : Memory  InitialCondition=1  InheritSampleTime=on
  t : ArgOut  DisableCoverage=on  ArgumentName=t
  wires:
  MMPP/5(lambda) -> Scope1/1
  D/1 -> MMPP/3("D ")
  MMPP/3(D) -> D/1
  Uniform Random Number/1 -> MMPP/5(rn)
  Constant/1 -> MMPP/4(M)
  MMPP/1(x) -> X/1
  MMPP/4(t) -> Scope/1, t/1
  MMPP/2(T) -> T/1
  T/1 -> MMPP/2("T ")
  X/1 -> MMPP/1("x ")

== system QueuingSys/Distro/MMPPArrivalTime14 ==
  MMPPArrivalTime : TriggerPort  TriggerType=function-call  IsSimulinkFunction=on  FunctionName=MMPPArrivalTime14  VariantControl=Variant
  Constant : Constant  Value=[0.0932806412615796 0.10475583265965 0.0293906242244008 0.77257290185437;0.471907175257639 0.0102399962080758 0.213294738374972 0.304558090159313;0.144664776062697 0.18890576566579 0.515159082839529 0.151270375431984;0.0444742945370317 0.0544987934264784 0.302642103523551 0.598384808512939]  SampleTime=-1
  D : Memory  InitialCondition=[0.0876437222952857;0.470425708481648]  InheritSampleTime=on
  MMPP : MATLAB Function  TreatAsAtomicUnit=on
  Scope : Scope
  Scope1 : Scope
  T : Memory  InitialCondition=[0 0.308204556021653]  InheritSampleTime=on
  Uniform Random Number : UniformRandomNumber  Minimum=0  Seed=randi(5000)
  X : Memory  InitialCondition=3  InheritSampleTime=on
  t : ArgOut  DisableCoverage=on  ArgumentName=t
  wires:
  MMPP/5(lambda) -> Scope1/1
  D/1 -> MMPP/3("D ")
  MMPP/3(D) -> D/1
  Uniform Random Number/1 -> MMPP/5(rn)
  Constant/1 -> MMPP/4(M)
  MMPP/1(x) -> X/1
  MMPP/4(t) -> Scope/1, t/1
  MMPP/2(T) -> T/1
  T/1 -> MMPP/2("T ")
  X/1 -> MMPP/1("x ")

== system QueuingSys/Distro/MMPPArrivalTime15 ==
  MMPPArrivalTime : TriggerPort  TriggerType=function-call  IsSimulinkFunction=on  FunctionName=MMPPArrivalTime15  VariantControl=Variant
  Constant : Constant  Value=[0.0401058375505951 0.0377051481145618 0.706069345359974 0.216119668974869;0.409640909389935 0.403089821424346 0.176283804311435 0.0109854648742844;0.252265741765676 0.485912128986102 0.103325925540027 0.158496203708196;0.166781547605669 0.463458590345799 0.226111139160036 0.143648722888496]  SampleTime=-1
  D : Memory  InitialCondition=[0.348220780592835;0.537149596656765]  InheritSampleTime=on
  MMPP : MATLAB Function  TreatAsAtomicUnit=on
  Scope : Scope
  Scope1 : Scope
  T : Memory  InitialCondition=[0 0.739455792730707]  InheritSampleTime=on
  Uniform Random Number : UniformRandomNumber  Minimum=0  Seed=randi(5000)
  X : Memory  InitialCondition=1  InheritSampleTime=on
  t : ArgOut  DisableCoverage=on  ArgumentName=t
  wires:
  MMPP/5(lambda) -> Scope1/1
  D/1 -> MMPP/3("D ")
  MMPP/3(D) -> D/1
  Uniform Random Number/1 -> MMPP/5(rn)
  Constant/1 -> MMPP/4(M)
  MMPP/1(x) -> X/1
  MMPP/4(t) -> Scope/1, t/1
  MMPP/2(T) -> T/1
  T/1 -> MMPP/2("T ")
  X/1 -> MMPP/1("x ")

== system QueuingSys/Distro/MMPPArrivalTime16 ==
  MMPPArrivalTime : TriggerPort  TriggerType=function-call  IsSimulinkFunction=on  FunctionName=MMPPArrivalTime16  VariantControl=Variant
  Constant : Constant  Value=[0.247126295403578 0.752873704596422;0.513365640214302 0.486634359785698]  SampleTime=-1
  D : Memory  InitialCondition=[0.719337934780301;0.0335931645744745]  InheritSampleTime=on
  MMPP : MATLAB Function  TreatAsAtomicUnit=on
  Scope : Scope
  Scope1 : Scope
  T : Memory  InitialCondition=[0 0.0257259796336265]  InheritSampleTime=on
  Uniform Random Number : UniformRandomNumber  Minimum=0  Seed=randi(5000)
  X : Memory  InitialCondition=1  InheritSampleTime=on
  t : ArgOut  DisableCoverage=on  ArgumentName=t
  wires:
  MMPP/5(lambda) -> Scope1/1
  D/1 -> MMPP/3("D ")
  MMPP/3(D) -> D/1
  Uniform Random Number/1 -> MMPP/5(rn)
  Constant/1 -> MMPP/4(M)
  MMPP/1(x) -> X/1
  MMPP/4(t) -> Scope/1, t/1
  MMPP/2(T) -> T/1
  T/1 -> MMPP/2("T ")
  X/1 -> MMPP/1("x ")

== system QueuingSys/Distro/MMPPArrivalTime17 ==
  MMPPArrivalTime : TriggerPort  TriggerType=function-call  IsSimulinkFunction=on  FunctionName=MMPPArrivalTime17  VariantControl=Variant
  Constant : Constant  Value=[0.142182067718587 0.10242319115561 0.0556781393969113 0.171330102856225 0.263541060784112 0.264845438088556;0.103054796463935 0.0101439592999038 0.0772887080596481 0.467031778718977 0.0217735045375128 0.320707252920024;0.357445245923076 0.130106801895566 0.193447848546424 0.166015947238577 0.0111891345566429 0.141795021839715;0.0976925190207533 0.135264618666977 0.178842475388613 0.244912620550516 0.202139587297631 0.141148179075509;0.574255189472711 0.0562080082118683 0.0310161428492547 0.00992666422381366 0.205097191159669 0.123496804082684;0.295186574288889 0.351084786761704 0.132939752996957 0.05525339538785 0.0794355868305393 0.0860999037340608]  SampleTime=-1
  D : Memory  InitialCondition=[0.921243055684344;0.781648862269082]  InheritSampleTime=on
  MMPP : MATLAB Function  TreatAsAtomicUnit=on
  Scope : Scope
  Scope1 : Scope
  T : Memory  InitialCondition=[0 1.39063680207556]  InheritSampleTime=on
  Uniform Random Number : UniformRandomNumber  Minimum=0  Seed=randi(5000)
  X : Memory  InitialCondition=6  InheritSampleTime=on
  t : ArgOut  DisableCoverage=on  ArgumentName=t
  wires:
  MMPP/5(lambda) -> Scope1/1
  D/1 -> MMPP/3("D ")
  MMPP/3(D) -> D/1
  Uniform Random Number/1 -> MMPP/5(rn)
  Constant/1 -> MMPP/4(M)
  MMPP/1(x) -> X/1
  MMPP/4(t) -> Scope/1, t/1
  MMPP/2(T) -> T/1
  T/1 -> MMPP/2("T ")
  X/1 -> MMPP/1("x ")

== system QueuingSys/Distro/MMPPArrivalTime18 ==
  MMPPArrivalTime : TriggerPort  TriggerType=function-call  IsSimulinkFunction=on  FunctionName=MMPPArrivalTime18  VariantControl=Variant
  Constant : Constant  Value=[0.36479369994344 0.462900226565751 0.17230607349081;0.476138543609568 0.316069483562708 0.207791972827724;0.141021621259036 0.374537492419174 0.484440886321789]  SampleTime=-1
  D : Memory  InitialCondition=[0.893525483138456;0.440476366658922]  InheritSampleTime=on
  MMPP : MATLAB Function  TreatAsAtomicUnit=on
  Scope : Scope
  Scope1 : Scope
  T : Memory  InitialCondition=[0 0.368844932281477]  InheritSampleTime=on
  Uniform Random Number : UniformRandomNumber  Minimum=0  Seed=randi(5000)
  X : Memory  InitialCondition=1  InheritSampleTime=on
  t : ArgOut  DisableCoverage=on  ArgumentName=t
  wires:
  MMPP/5(lambda) -> Scope1/1
  D/1 -> MMPP/3("D ")
  MMPP/3(D) -> D/1
  Uniform Random Number/1 -> MMPP/5(rn)
  Constant/1 -> MMPP/4(M)
  MMPP/1(x) -> X/1
  MMPP/4(t) -> Scope/1, t/1
  MMPP/2(T) -> T/1
  T/1 -> MMPP/2("T ")
  X/1 -> MMPP/1("x ")

== system QueuingSys/Distro/MMPPArrivalTime19 ==
  MMPPArrivalTime : TriggerPort  TriggerType=function-call  IsSimulinkFunction=on  FunctionName=MMPPArrivalTime19  VariantControl=Variant
  Constant : Constant  Value=[0.100196380161333 0.183988141823339 0.233315176767858 0.217391823256139 0.261557959711383 0.00355051827994898;0.114873126785534 0.00714140737218188 0.361231527053543 0.290640497638917 0.189285737434527 0.0368277037152965;0.321199797540799 0.197489564932846 0.0042361522573353 0.108889605662573 0.156903996816323 0.211280882790124;0.0340436276249291 0.178122298500438 0.204603153730884 0.150518564386135 0.219004712210613 0.213707643547001;0.239025989728612 0.204743324164089 0.0100553117822104 0.260798925131623 0.207805299304363 0.0775711498891029;0.190675972933525 0.197843245764607 0.114296484011605 0.142435196647194 0.183015006763999 0.17173409387907]  SampleTime=-1
  D : Memory  InitialCondition=[0.725059755063973;0.894647612386255]  InheritSampleTime=on
  MMPP : MATLAB Function  TreatAsAtomicUnit=on
  Scope : Scope
  Scope1 : Scope
  T : Memory  InitialCondition=[0 1.91171080369443]  InheritSampleTime=on
  Uniform Random Number : UniformRandomNumber  Minimum=0  Seed=randi(5000)
  X : Memory  InitialCondition=4  InheritSampleTime=on
  t : ArgOut  DisableCoverage=on  ArgumentName=t
  wires:
  MMPP/5(lambda) -> Scope1/1
  D/1 -> MMPP/3("D ")
  MMPP/3(D) -> D/1
  Uniform Random Number/1 -> MMPP/5(rn)
  Constant/1 -> MMPP/4(M)
  MMPP/1(x) -> X/1
  MMPP/4(t) -> Scope/1, t/1
  MMPP/2(T) -> T/1
  T/1 -> MMPP/2("T ")
  X/1 -> MMPP/1("x ")

== system QueuingSys/Distro/MMPPArrivalTime2 ==
  MMPPArrivalTime : TriggerPort  TriggerType=function-call  IsSimulinkFunction=on  FunctionName=MMPPArrivalTime2  VariantControl=Variant
  Constant : Constant  Value=[0.15884192538535 0.133998619253844 0.192861537573911 0.0729540272391441 0.0839832034460873 0.218327275040528 0.139033412061137;0.292168908641615 0.25713089494532 0.0244750220648784 0.0288494700150006 0.0405950667340419 0.201826086790309 0.154954550808835;0.222124589291749 0.11134546054113 0.102483839110111 0.173300002319679 0.0879375893788136 0.202988833464514 0.0998196858940033;0.136813135990492 0.077088788143117 0.228272549387912 0.145672318507039 0.158737691331221 0.195747178916856 0.0576683377233621;0.227910842207971 0.0690468360880319 0.186408934184888 0.199257851488995 0.147196140052964 0.0809149588283843 0.0892644371487658;0.240119078057207 0.113321752510841 0.120000413050052 0.132523073084235 0.218861066104953 0.173160128962805 0.00201448822990683;0.139811643327977 0.00493429103793756 0.0261590050915976 0.123454384657263 0.223097236304063 0.181581676843822 0.30096176273734]  SampleTime=-1
  D : Memory  InitialCondition=[0.891845693826279;0.420824840285832]  InheritSampleTime=on
  MMPP : MATLAB Function  TreatAsAtomicUnit=on
  Scope : Scope
  Scope1 : Scope
  T : Memory  InitialCondition=[0 0.465759106178831]  InheritSampleTime=on
  Uniform Random Number : UniformRandomNumber  Minimum=0  Seed=randi(5000)
  X : Memory  InitialCondition=5  InheritSampleTime=on
  t : ArgOut  DisableCoverage=on  ArgumentName=t
  wires:
  MMPP/5(lambda) -> Scope1/1
  D/1 -> MMPP/3("D ")
  MMPP/3(D) -> D/1
  Uniform Random Number/1 -> MMPP/5(rn)
  Constant/1 -> MMPP/4(M)
  MMPP/1(x) -> X/1
  MMPP/4(t) -> Scope/1, t/1
  MMPP/2(T) -> T/1
  T/1 -> MMPP/2("T ")
  X/1 -> MMPP/1("x ")

== system QueuingSys/Distro/MMPPArrivalTime20 ==
  MMPPArrivalTime : TriggerPort  TriggerType=function-call  IsSimulinkFunction=on  FunctionName=MMPPArrivalTime20  VariantControl=Variant
  Constant : Constant  Value=[0.12449012260309 0.219639323364643 0.203904836796487 0.192899163233864 0.13923187971756 0.106169819348564 0.0136648549357922;0.148783753698043 0.131894050354901 0.261202026969907 0.193714960515092 0.210339933427074 0.0367602390366614 0.0173050359983226;0.0665705962732076 0.221271145990759 0.0742463040564804 0.237682762652747 0.226697428451229 0.16659146001069 0.00694030256488681;0.210181303581902 0.131988108019088 0.0327051200797571 0.186352901896909 0.0821670514863853 0.220941567740386 0.135663947195573;0.285886442069194 0.150757423230573 4.60305561039838e-05 0.0585220556187974 0.160808385569082 0.148439869538163 0.195539793418086;0.00841096195551623 0.0124009387818189 0.161375906151959 0.489270970759982 0.0847006986737151 0.08924786000313 0.154592663673878;0.140728112778285 0.149517809963565 0.157150887569631 0.103243684820997 0.138261433388978 0.087422821338706 0.223675250139838]  SampleTime=-1
  D : Memory  InitialCondition=[0.939838254337713;0.485154691181415]  InheritSampleTime=on
  MMPP : MATLAB Function  TreatAsAtomicUnit=on
  Scope : Scope
  Scope1 : Scope
  T : Memory  InitialCondition=[0 0.557129909397452]  InheritSampleTime=on
  Uniform Random Number : UniformRandomNumber  Minimum=0  Seed=randi(5000)
  X : Memory  InitialCondition=5  InheritSampleTime=on
  t : ArgOut  DisableCoverage=on  ArgumentName=t
  wires:
  MMPP/5(lambda) -> Scope1/1
  D/1 -> MMPP/3("D ")
  MMPP/3(D) -> D/1
  Uniform Random Number/1 -> MMPP/5(rn)
  Constant/1 -> MMPP/4(M)
  MMPP/1(x) -> X/1
  MMPP/4(t) -> Scope/1, t/1
  MMPP/2(T) -> T/1
  T/1 -> MMPP/2("T ")
  X/1 -> MMPP/1("x ")

== system QueuingSys/Distro/MMPPArrivalTime21 ==
  MMPPArrivalTime : TriggerPort  TriggerType=function-call  IsSimulinkFunction=on  FunctionName=MMPPArrivalTime21  VariantControl=Variant
  Constant : Constant  Value=[0.0995429072257098 0.343063782981496 0.278166311492051 0.0300623165189305 0.249164681781813;0.437115128328776 0.02823995206027 0.141763895114891 0.346653839377337 0.0462271851187261;0.114825822328873 0.253346401353542 0.153202910993701 0.159291408951949 0.319333456371934;0.263249973276382 0.0433788645375475 0.331575601744002 0.0524415216515974 0.309354038790471;0.0643783589567225 0.396260037204926 0.204517786121284 0.312172709115031 0.0226711086020365]  SampleTime=-1
  D : Memory  InitialCondition=[0.889264629794461;0.347723192695842]  InheritSampleTime=on
  MMPP : MATLAB Function  TreatAsAtomicUnit=on
  Scope : Scope
  Scope1 : Scope
  T : Memory  InitialCondition=[0 0.404878714622579]  InheritSampleTime=on
  Uniform Random Number : UniformRandomNumber  Minimum=0  Seed=randi(5000)
  X : Memory  InitialCondition=4  InheritSampleTime=on
  t : ArgOut  DisableCoverage=on  ArgumentName=t
  wires:
  MMPP/5(lambda) -> Scope1/1
  D/1 -> MMPP/3("D ")
  MMPP/3(D) -> D/1
  Uniform Random Number/1 -> MMPP/5(rn)
  Constant/1 -> MMPP/4(M)
  MMPP/1(x) -> X/1
  MMPP/4(t) -> Scope/1, t/1
  MMPP/2(T) -> T/1
  T/1 -> MMPP/2("T ")
  X/1 -> MMPP/1("x ")

== system QueuingSys/Distro/MMPPArrivalTime22 ==
  MMPPArrivalTime : TriggerPort  TriggerType=function-call  IsSimulinkFunction=on  FunctionName=MMPPArrivalTime22  VariantControl=Variant
  Constant : Constant  Value=[0.135952733360217 0.0481795179297998 0.1860133957593 0.130251076994528 0.178219532167928 0.321383743788227;0.097938354168561 0.198746041737789 0.0708168116692911 0.0978570854606238 0.239433206513901 0.295208500449834;0.0543097649214826 0.108744059482257 0.351752252521196 0.215050996284466 0.136942432180333 0.133200494610265;0.21867731987028 0.131601762433815 0.179080327813011 0.206182697784302 0.245995643539454 0.0184622485591375;0.095474184110026 0.178545516846053 0.0384095217937662 0.155708126481729 0.248546098505247 0.283316552263179;0.408334218482528 0.0234309858594646 0.161576879504063 0.355469306966104 0.00879608044233515 0.0423925287455048]  SampleTime=-1
  D : Memory  InitialCondition=[0.915525126570028;0.522011578805557]  InheritSampleTime=on
  MMPP : MATLAB Function  TreatAsAtomicUnit=on
  Scope : Scope
  Scope1 : Scope
  T : Memory  InitialCondition=[0 0.585971141761207]  InheritSampleTime=on
  Uniform Random Number : UniformRandomNumber  Minimum=0  Seed=randi(5000)
  X : Memory  InitialCondition=4  InheritSampleTime=on
  t : ArgOut  DisableCoverage=on  ArgumentName=t
  wires:
  MMPP/5(lambda) -> Scope1/1
  D/1 -> MMPP/3("D ")
  MMPP/3(D) -> D/1
  Uniform Random Number/1 -> MMPP/5(rn)
  Constant/1 -> MMPP/4(M)
  MMPP/1(x) -> X/1
  MMPP/4(t) -> Scope/1, t/1
  MMPP/2(T) -> T/1
  T/1 -> MMPP/2("T ")
  X/1 -> MMPP/1("x ")

== system QueuingSys/Distro/MMPPArrivalTime23 ==
  MMPPArrivalTime : TriggerPort  TriggerType=function-call  IsSimulinkFunction=on  FunctionName=MMPPArrivalTime23  VariantControl=Variant
  Constant : Constant  Value=[0.701149545955533 0.298850454044467;0.214492260068378 0.785507739931622]  SampleTime=-1
  D : Memory  InitialCondition=[0.662215360447538;0.10708839955975]  InheritSampleTime=on
  MMPP : MATLAB Function  TreatAsAtomicUnit=on
  Scope : Scope
  Scope1 : Scope
  T : Memory  InitialCondition=[0 0.0242950438233376]  InheritSampleTime=on
  Uniform Random Number : UniformRandomNumber  Minimum=0  Seed=randi(5000)
  X : Memory  InitialCondition=2  InheritSampleTime=on
  t : ArgOut  DisableCoverage=on  ArgumentName=t
  wires:
  MMPP/5(lambda) -> Scope1/1
  D/1 -> MMPP/3("D ")
  MMPP/3(D) -> D/1
  Uniform Random Number/1 -> MMPP/5(rn)
  Constant/1 -> MMPP/4(M)
  MMPP/1(x) -> X/1
  MMPP/4(t) -> Scope/1, t/1
  MMPP/2(T) -> T/1
  T/1 -> MMPP/2("T ")
  X/1 -> MMPP/1("x ")
